simulink model "Simulink_Model"  (R2023a)
settings: Solver=VariableStepAuto  StartTime=0.0  StopTime=10.0  RelTol=1e-3
undefined symbols (not defined in the file or in its folder): aoa, Earth, gustU_pert, gustV_pert, gustW_pert, InConds, mach, rocketAeroDatabase, WGS84
libraries: aerolibatmos2 x2, aerolibwind2 x1, aerolibtransform2 x1
settings Model: Creator=cnsyk  LastModifiedBy=cnsyk

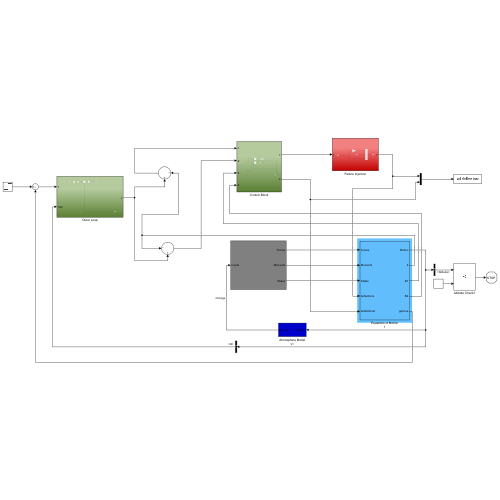
[thumbnail: Simulink's stored preview of the top-level diagram]
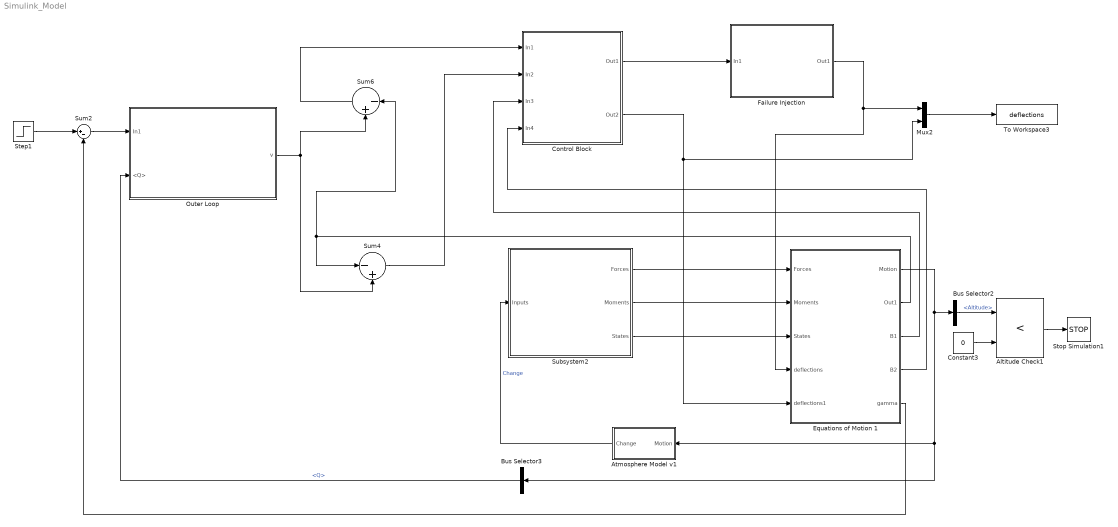
== system Simulink_Model ==
  Altitude Check1 : RelationalOperator  Operator=<  OutDataTypeStr=boolean  RndMeth=Simplest  InputSameDT=off
  Atmosphere Model v1 : Subsystem
  Bus Selector2 : BusSelector  OutputSignals=Altitude
  Bus Selector3 : BusSelector  OutputSignals=Q
  Constant3 : Constant  Value=0
  Control Block : Subsystem
  Equations of Motion 1 : Subsystem
  Failure Injection : Subsystem
  Mux2 : Mux  Inputs=2
  Outer Loop : Subsystem
  Step1 : Step  Time=0  After=deg2rad(80)  SampleTime=0
  Stop Simulation1 : Stop
  Subsystem2 : Subsystem
  Sum2 : Sum  Inputs=|+-
  Sum4 : Sum  Inputs=|-+
  Sum6 : Sum  Inputs=|-+
  To Workspace3 : ToWorkspace  VariableName=deflections  SampleTime=-1
  wires:
  Constant3/1 -> Altitude Check1/2
  Equations of Motion 1/2(Out1) -> Sum4/1, Sum6/1
  Subsystem2/3(States) -> Equations of Motion 1/3(States)
  Subsystem2/2(Moments) -> Equations of Motion 1/2("Moments ")
  Subsystem2/1(Forces) -> Equations of Motion 1/1("Forces ")
  Equations of Motion 1/5(gamma) -> Sum2/2
  Bus Selector2/1 -> Altitude Check1/1  "<Altitude>"
  Altitude Check1/1 -> Stop Simulation1/1
  Step1/1 -> Sum2/1
  Mux2/1 -> To Workspace3/1
  Equations of Motion 1/1(Motion) -> Atmosphere Model v1/1("Motion "), Bus Selector3/1, Bus Selector2/1
  Atmosphere Model v1/1(Change) -> Subsystem2/1("Inputs ")  "Change"
  Control Block/2(Out2) -> Mux2/2, Equations of Motion 1/5(deflections1)
  Sum6/1 -> Control Block/1(In1)
  Sum4/1 -> Control Block/2(In2)
  Equations of Motion 1/3(B1) -> Control Block/3(In3)
  Equations of Motion 1/4(B2) -> Control Block/4(In4)
  Failure Injection/1(Out1) -> Equations of Motion 1/4(deflections), Mux2/1
  Control Block/1(Out1) -> Failure Injection/1(In1)
  Outer Loop/1(v) -> Sum4/2, Sum6/2
  Sum2/1 -> Outer Loop/1(In1)
  Bus Selector3/1 -> Outer Loop/2(<Q>)  "<Q>"

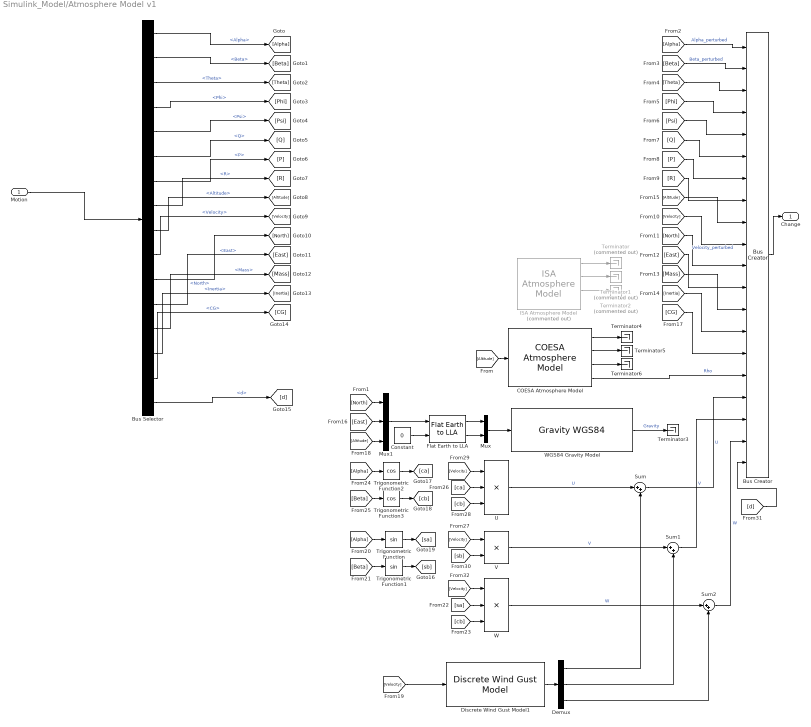
== system Simulink_Model/Atmosphere Model v1 ==
  "Motion " : Inport
  Bus Creator : BusCreator  Inputs=20
  Bus Selector : BusSelector  OutputSignals=Alpha,Beta,Theta,Phi,Psi,Q,P,R,Altitude,Velocity,North,East,Mass,Inertia,CG,d
  COESA Atmosphere Model : aerolibatmos2/COESA Atmosphere Model  units=Metric (MKS)  spec=1976 COESA-extended U.S. Standard Atmosphere  model=Profile  profile_var=High temperature  profile_percent=1%  profile_alt=5 km (16404 ft)  envelope_var=High temperature  envelope_percent=1%  action=Warning
  Constant : Constant  Value=0
  Demux : Demux  Outputs=3
  Discrete Wind Gust Model1 : aerolibwind2/Discrete Wind Gust Model  units=Metric (MKS)  Gx=on  Gy=on  Gz=on  t_0=5  d_m=[120 120 80]  v_m=[gustU_pert gustV_pert gustW_pert]
  Flat Earth to LLA : aerolibtransform2/Flat Earth to LLA  units=Metric (MKS)  ptype=Earth (WGS84)  F=1/298.257223563  R=6378137  refPosPort=off  LL0=[0 10]  psi=0
  ISA Atmosphere Model : aerolibatmos2/ISA Atmosphere Model  Commented=on  custom=off  g=9.80665  gamma=1.4  R=287.0531  L=0.0065  h_trop=11000  h_strat=20000  rho0=1.225  P0=101325  T0=288.15  h0=0
  Mux : Mux  Inputs=2
  Mux1 : Mux  Inputs=3
  Sum : Sum  Inputs=|++
  Sum1 : Sum  Inputs=|++
  Sum2 : Sum  Inputs=|++
  Terminator : Terminator  Commented=on
  Terminator1 : Terminator  Commented=on
  Terminator2 : Terminator  Commented=on
  Terminator{3..6} (4 alike) : Terminator
  Trigonometric Function : Trigonometry
  Trigonometric Function1 : Trigonometry
  Trigonometric Function2 : Trigonometry  Operator=cos
  Trigonometric Function3 : Trigonometry  Operator=cos
  U : Product  Inputs=3
  V : Product
  W : Product  Inputs=3
  "WGS84 Gravity Model  " : GravityWGS84
  Change : Outport  VectorParamsAs1DForOutWhenUnconnected=off
  wires:
  V/1 -> Sum1/1  "V"
  [Q] -> Bus Creator/6
  [ca] -> U/2
  [Phi] -> Bus Creator/4
  [R] -> Bus Creator/8
  [East] -> Bus Creator/12
  Bus Selector/5 -> [Psi]  "<Psi>"
  W/1 -> Sum2/1  "W"
  [Velocity] -> U/1
  [Theta] -> Bus Creator/3
  [sa] -> W/2
  Sum1/1 -> Bus Creator/18  "V"
  [sb] -> V/2
  U/1 -> Sum/1  "U"
  [North] -> Bus Creator/11
  Sum2/1 -> Bus Creator/19  "W"
  [Velocity] -> W/1
  [Altitude] -> Mux1/3
  Trigonometric Function/1 -> [sa]
  Mux/1 -> "WGS84 Gravity Model  "/1
  Bus Selector/7 -> [P]  "<P>"
  [Mass] -> Bus Creator/13
  [cb] -> U/3
  Trigonometric Function2/1 -> [ca]
  [cb] -> W/3
  Demux/2 -> Sum1/2
  [Altitude] -> Bus Creator/9
  Bus Selector/15 -> [CG]  "<CG>"
  ISA Atmosphere Model/2 -> Terminator1/1
  [Beta] -> Trigonometric Function3/1
  Discrete Wind Gust Model1/1 -> Demux/1
  [CG] -> Bus Creator/15
  Bus Selector/1 -> [Alpha]  "<Alpha>"
  [Alpha] -> Trigonometric Function/1
  [Beta] -> Bus Creator/2  "Beta_perturbed"
  Demux/3 -> Sum2/2
  [Beta] -> Trigonometric Function1/1
  "Motion "/1 -> Bus Selector/1
  [Velocity] -> Bus Creator/10  "Velocity_perturbed"
  Bus Selector/8 -> [R]  "<R>"
  Sum/1 -> Bus Creator/17  "U"
  Bus Selector/2 -> [Beta]  "<Beta>"
  Bus Selector/6 -> [Q]  "<Q>"
  "WGS84 Gravity Model  "/1 -> Terminator3/1  "Gravity"
  Mux1/1 -> Flat Earth to LLA/1
  Bus Selector/9 -> [Altitude]  "<Altitude>"
  [P] -> Bus Creator/7
  [East] -> Mux1/2
  [Velocity] -> Discrete Wind Gust Model1/1
  Bus Selector/14 -> [Inertia]  "<Inertia>"
  Bus Selector/10 -> [Velocity]  "<Velocity>"
  Trigonometric Function1/1 -> [sb]
  [Inertia] -> Bus Creator/14
  Bus Selector/11 -> [North]  "<North>"
  Trigonometric Function3/1 -> [cb]
  Bus Selector/4 -> [Phi]  "<Phi>"
  Bus Selector/12 -> [East]  "<East>"
  Bus Selector/3 -> [Theta]  "<Theta>"
  [Alpha] -> Bus Creator/1  "Alpha_perturbed"
  [Psi] -> Bus Creator/5
  Constant/1 -> Flat Earth to LLA/2
  [North] -> Mux1/1
  Bus Creator/1 -> Change/1
  ISA Atmosphere Model/1 -> Terminator/1
  Flat Earth to LLA/1 -> Mux/1
  Demux/1 -> Sum/2
  Bus Selector/13 -> [Mass]  "<Mass>"
  [Velocity] -> V/1
  ISA Atmosphere Model/3 -> Terminator2/1
  [Alpha] -> Trigonometric Function2/1
  Flat Earth to LLA/2 -> Mux/2
  [Altitude] -> COESA Atmosphere Model/1
  COESA Atmosphere Model/1 -> Terminator4/1
  COESA Atmosphere Model/2 -> Terminator5/1
  COESA Atmosphere Model/3 -> Terminator6/1
  COESA Atmosphere Model/4 -> Bus Creator/16  "Rho"
  Bus Selector/16 -> [d]  "<d>"
  [d] -> Bus Creator/20

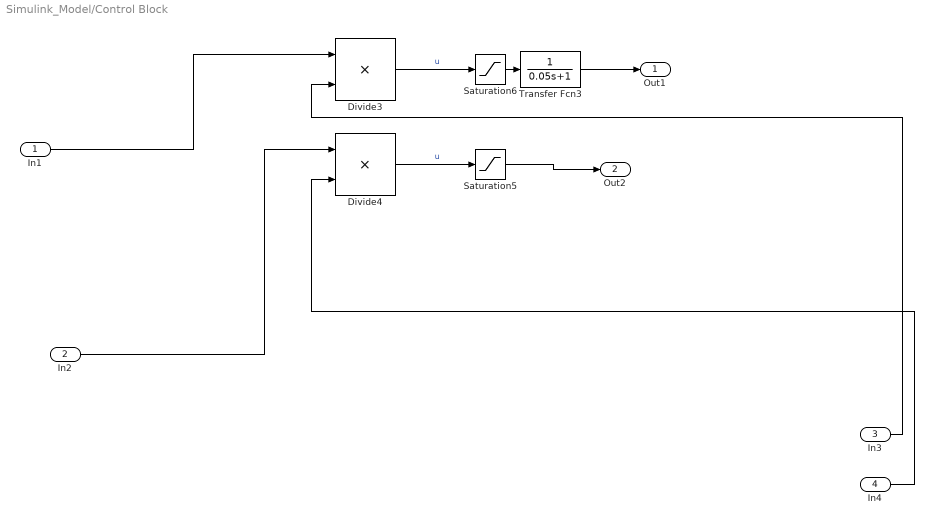
== system Simulink_Model/Control Block ==
  In1 : Inport
  In2 : Inport  Port=2
  In3 : Inport  Port=3
  In4 : Inport  Port=4
  Divide3 : Product  Inputs=**
  Divide4 : Product  Inputs=**
  Saturation5 : Saturate  UpperLimit=deg2rad(5)  LowerLimit=-deg2rad(5)
  Saturation6 : Saturate  UpperLimit=deg2rad(5)  LowerLimit=-deg2rad(5)
  Transfer Fcn3 : TransferFcn  Denominator=[0.05 1]
  Out1 : Outport
  Out2 : Outport  Port=2
  wires:
  In3/1 -> Divide3/2
  In4/1 -> Divide4/2
  Saturation5/1 -> Out2/1
  Saturation6/1 -> Transfer Fcn3/1
  Divide3/1 -> Saturation6/1  "u"
  Divide4/1 -> Saturation5/1  "u"
  In2/1 -> Divide4/1
  In1/1 -> Divide3/1
  Transfer Fcn3/1 -> Out1/1

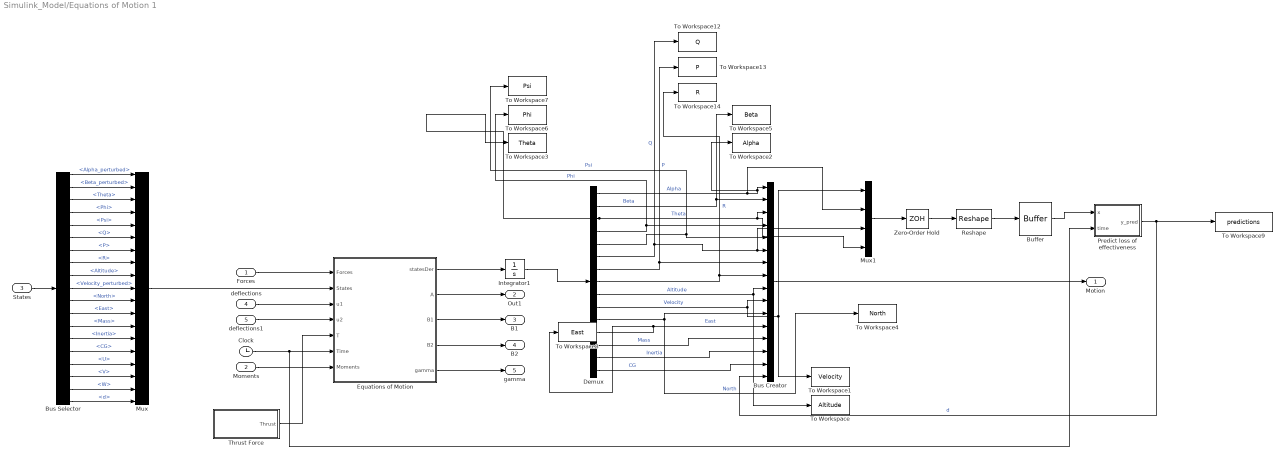
== system Simulink_Model/Equations of Motion 1 ==
  "Forces " : Inport
  "Moments " : Inport  Port=2
  States : Inport  Port=3
  deflections : Inport  Port=4
  deflections1 : Inport  Port=5
  Buffer : Buffer  N=20  V=19  OutputFrames=off
  Bus Creator : BusCreator  Inputs=16
  Bus Selector : BusSelector  OutputSignals=Alpha_perturbed,Beta_perturbed,Theta,Phi,Psi,Q,P,R,Altitude,Velocity_perturbed,North,East,Mass,Inertia,CG,U,V,W,d
  Clock : Clock
  Demux : Demux  Outputs=15
  Equations of Motion : MATLAB Function  TreatAsAtomicUnit=on
  Integrator1 : Integrator  InitialCondition=InConds
  Mux : Mux  Inputs=19
  Mux1 : Mux
  Predict loss of effectiveness : MATLAB Function  TreatAsAtomicUnit=on
  Reshape : Reshape  OutputDimensionality=Customize  OutputDimensions=[1,4]
  "Thrust Force " : Subsystem
  To Workspace : ToWorkspace  VariableName=Altitude  SampleTime=-1
  To Workspace1 : ToWorkspace  VariableName=Velocity  SampleTime=-1
  To Workspace12 : ToWorkspace  VariableName=Q  SampleTime=-1
  To Workspace13 : ToWorkspace  VariableName=P  SampleTime=-1
  To Workspace14 : ToWorkspace  VariableName=R  SampleTime=-1
  To Workspace2 : ToWorkspace  VariableName=Alpha  SampleTime=-1
  To Workspace3 : ToWorkspace  VariableName=Theta  SampleTime=-1
  To Workspace4 : ToWorkspace  VariableName=North  SampleTime=-1
  To Workspace5 : ToWorkspace  VariableName=Beta  SampleTime=-1
  To Workspace6 : ToWorkspace  VariableName=Phi  SampleTime=-1
  To Workspace7 : ToWorkspace  VariableName=Psi  SampleTime=-1
  To Workspace8 : ToWorkspace  VariableName=East  SampleTime=-1
  To Workspace9 : ToWorkspace  VariableName=predictions  SampleTime=-1
  Zero-Order Hold : ZeroOrderHold  SampleTime=-1
  Motion : Outport  VectorParamsAs1DForOutWhenUnconnected=off
  Out1 : Outport  Port=2
  B1 : Outport  Port=3
  B2 : Outport  Port=4
  gamma : Outport  Port=5
  wires:
  "Moments "/1 -> Equations of Motion/7(Moments)
  "Forces "/1 -> Equations of Motion/1(Forces)
  Demux/10 -> Bus Creator/10, To Workspace1/1, Mux1/1  "Velocity"
  Demux/9 -> Bus Creator/9, To Workspace/1  "Altitude"
  Demux/8 -> To Workspace14/1, Bus Creator/8  "R"
  Demux/7 -> To Workspace13/1, Bus Creator/7  "P"
  Demux/6 -> Mux1/3, Bus Creator/6, To Workspace12/1  "Q"
  Demux/5 -> To Workspace7/1, Bus Creator/5  "Psi"
  Demux/4 -> To Workspace6/1, Bus Creator/4  "Phi"
  Demux/3 -> Mux1/4, Bus Creator/3, To Workspace3/1  "Theta"
  Bus Creator/1 -> Motion/1
  Demux/11 -> To Workspace4/1, Bus Creator/11  "North"
  Demux/12 -> To Workspace8/1, Bus Creator/12  "East"
  Demux/13 -> Bus Creator/13  "Mass"
  Demux/14 -> Bus Creator/14  "Inertia"
  Demux/15 -> Bus Creator/15  "CG"
  States/1 -> Bus Selector/1
  Mux/1 -> Equations of Motion/2(States)
  Clock/1 -> Equations of Motion/6(Time), Predict loss of effectiveness/2(time)
  Bus Selector/1 -> Mux/1  "<Alpha_perturbed>"
  Bus Selector/5 -> Mux/5  "<Psi>"
  Bus Selector/4 -> Mux/4  "<Phi>"
  Bus Selector/3 -> Mux/3  "<Theta>"
  Bus Selector/2 -> Mux/2  "<Beta_perturbed>"
  Demux/1 -> Mux1/2, Bus Creator/1, To Workspace2/1  "Alpha"
  Demux/2 -> To Workspace5/1, Bus Creator/2  "Beta"
  Bus Selector/6 -> Mux/6  "<Q>"
  Bus Selector/7 -> Mux/7  "<P>"
  Bus Selector/8 -> Mux/8  "<R>"
  Bus Selector/9 -> Mux/9  "<Altitude>"
  Bus Selector/14 -> Mux/14  "<Inertia>"
  Bus Selector/13 -> Mux/13  "<Mass>"
  Bus Selector/12 -> Mux/12  "<East>"
  Bus Selector/11 -> Mux/11  "<North>"
  Bus Selector/10 -> Mux/10  "<Velocity_perturbed>"
  Bus Selector/15 -> Mux/15  "<CG>"
  Bus Selector/17 -> Mux/17  "<V>"
  Bus Selector/16 -> Mux/16  "<U>"
  Bus Selector/18 -> Mux/18  "<W>"
  deflections/1 -> Equations of Motion/3(u1)
  Equations of Motion/3(B1) -> B1/1
  Equations of Motion/2(A) -> Out1/1
  "Thrust Force "/1(Thrust) -> Equations of Motion/5(T)
  Equations of Motion/5(gamma) -> gamma/1
  Integrator1/1 -> Demux/1
  deflections1/1 -> Equations of Motion/4(u2)
  Equations of Motion/4(B2) -> B2/1
  Equations of Motion/1(statesDer) -> Integrator1/1
  Reshape/1 -> Buffer/1
  Buffer/1 -> Predict loss of effectiveness/1(x)
  Predict loss of effectiveness/1(y_pred) -> To Workspace9/1, Bus Creator/16  "d"
  Mux1/1 -> Zero-Order Hold/1
  Zero-Order Hold/1 -> Reshape/1
  Bus Selector/19 -> Mux/19  "<d>"

== system Simulink_Model/Failure Injection ==
  In1 : Inport
  Clock2 : Clock
  Gain4 : Gain
  Switch2 : Switch  Criteria=u2 > Threshold  Threshold=6  SaturateOnIntegerOverflow=off  InputSameDT=off
  Out1 : Outport
  wires:
  In1/1 -> Switch2/3, Gain4/1
  Gain4/1 -> Switch2/1
  Clock2/1 -> Switch2/2
  Switch2/1 -> Out1/1

== system Simulink_Model/Outer Loop ==
  In1 : Inport
  <Q> : Inport  Port=2
  Delay2 : Delay  DelayLength=3  InitialCondition=0
  Gain2 : Gain  Gain=5
  Gain3 : Gain  Gain=10
  Saturation4 : Saturate  UpperLimit=deg2rad(5)  LowerLimit=-deg2rad(5)
  Sum5 : Sum  Inputs=|+-
  v : Outport
  wires:
  Delay2/1 -> Saturation4/1
  Gain3/1 -> v/1  "v"
  Gain2/1 -> Delay2/1
  <Q>/1 -> Sum5/2
  In1/1 -> Gain2/1
  Sum5/1 -> Gain3/1
  Saturation4/1 -> Sum5/1

== system Simulink_Model/Subsystem2 ==
  "Inputs " : Inport
  Moment Calculation : Subsystem
  Mux : Mux  Inputs=3
  Mux1 : Mux  Inputs=3
  Subsystem1 : Subsystem
  Forces : Outport  VectorParamsAs1DForOutWhenUnconnected=off
  Moments : Outport  Port=2  VectorParamsAs1DForOutWhenUnconnected=off
  States : Outport  Port=3  VectorParamsAs1DForOutWhenUnconnected=off
  wires:
  "Inputs "/1 -> Subsystem1/1("Inputs "), States/1, Moment Calculation/1("Inputs ")
  Moment Calculation/1("MCm ") -> Mux1/1
  Moment Calculation/2(MCl) -> Mux1/2
  Subsystem1/3(FCY) -> Mux/3
  Mux/1 -> Forces/1
  Subsystem1/1(FCL) -> Mux/1
  Mux1/1 -> Moments/1
  Subsystem1/2(FCD) -> Mux/2
  Moment Calculation/3(MCn) -> Mux1/3

== system Simulink_Model/Equations of Motion 1/Thrust Force  ==
  Clock : Clock
  If : If  IfExpression=u1 < 33
  If Action Subsystem : Subsystem  TreatAsAtomicUnit=on
  If Action Subsystem1 : Subsystem  TreatAsAtomicUnit=on
  Scope : Scope
  Sum : Sum  Inputs=+|+
  To Workspace : ToWorkspace  VariableName=thrust  SampleTime=-1
  Thrust : Outport  VectorParamsAs1DForOutWhenUnconnected=off
  wires:
  Sum/1 -> To Workspace/1, Thrust/1
  Clock/1 -> If Action Subsystem1/1(Time), If Action Subsystem/1(Time), If/1
  If/1 -> If Action Subsystem/Action
  If Action Subsystem/1(Thrust) -> Scope/1, Sum/1
  If/2 -> If Action Subsystem1/Action
  If Action Subsystem1/1(Thrust) -> Sum/2

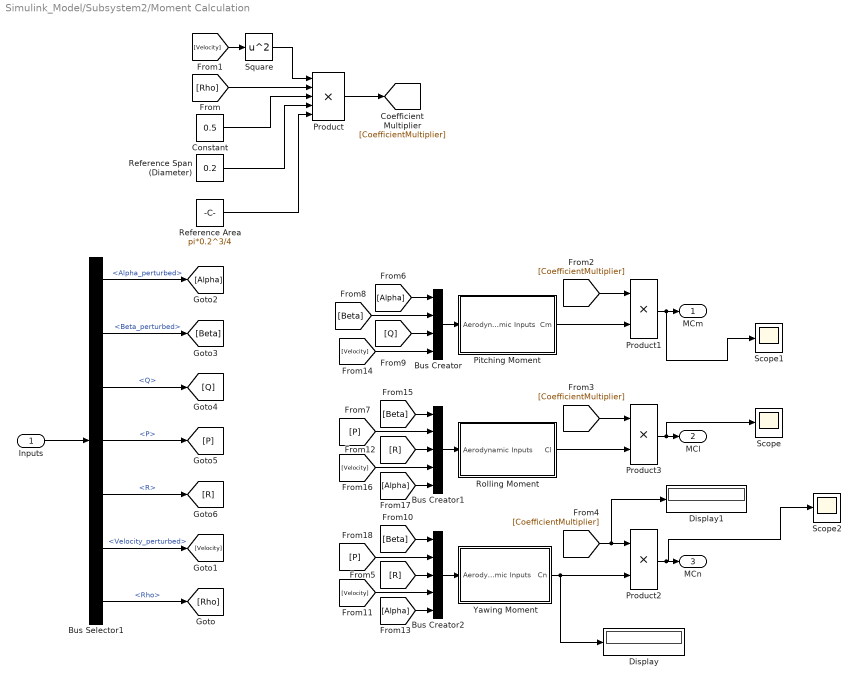
== system Simulink_Model/Subsystem2/Moment Calculation ==
  "Inputs " : Inport
  Bus Creator : BusCreator  Inputs=4
  Bus Creator1 : BusCreator  Inputs=5
  Bus Creator2 : BusCreator  Inputs=5
  Bus Selector1 : BusSelector  OutputSignals=Alpha_perturbed,Beta_perturbed,Q,P,R,Velocity_perturbed,Rho
  Constant : Constant  Value=0.5
  Display : Display
  Display1 : Display
  Pitching Moment : Subsystem
  Product : Product  Inputs=5
  Product1 : Product
  Product2 : Product
  Product3 : Product
  Reference Area : Constant  Value=pi*0.2^3/4
  Reference Span (Diameter) : Constant  Value=0.2
  Rolling Moment : Subsystem
  Scope : Scope
  Scope1 : Scope
  Scope2 : Scope
  Square : Math  Operator=square  SignedPower=on
  Yawing Moment : Subsystem
  "MCm " : Outport  VectorParamsAs1DForOutWhenUnconnected=off
  MCl : Outport  Port=2  VectorParamsAs1DForOutWhenUnconnected=off
  MCn : Outport  Port=3  VectorParamsAs1DForOutWhenUnconnected=off
  wires:
  Bus Selector1/4 -> [P]  "<P>"
  Bus Selector1/3 -> [Q]  "<Q>"
  Bus Selector1/5 -> [R]  "<R>"
  Bus Selector1/1 -> [Alpha]  "<Alpha_perturbed>"
  Bus Selector1/2 -> [Beta]  "<Beta_perturbed>"
  Product1/1 -> Scope1/1, "MCm "/1
  Product/1 -> [CoefficientMultiplier]
  [Velocity] -> Square/1
  [CoefficientMultiplier] -> Product1/1
  Reference Span (Diameter)/1 -> Product/4
  Bus Selector1/7 -> [Rho]  "<Rho>"
  Product3/1 -> Scope/1, MCl/1
  [CoefficientMultiplier] -> Display1/1, Product2/1
  [CoefficientMultiplier] -> Product3/1
  Bus Selector1/6 -> [Velocity]  "<Velocity_perturbed>"
  [Rho] -> Product/2
  "Inputs "/1 -> Bus Selector1/1
  Square/1 -> Product/1
  Constant/1 -> Product/3
  Bus Creator/1 -> Pitching Moment/1(Aerodynamic Inputs)
  [Alpha] -> Bus Creator/1
  [Q] -> Bus Creator/3
  [Beta] -> Bus Creator/2
  Bus Creator1/1 -> Rolling Moment/1(Aerodynamic Inputs)
  [Beta] -> Bus Creator1/1
  [P] -> Bus Creator1/2
  [R] -> Bus Creator1/3
  [Velocity] -> Bus Creator1/4
  Bus Creator2/1 -> Yawing Moment/1(Aerodynamic Inputs)
  Yawing Moment/1(Cn) -> Display/1, Product2/2
  [Velocity] -> Bus Creator/4
  [Alpha] -> Bus Creator1/5
  [P] -> Bus Creator2/2
  [Velocity] -> Bus Creator2/4
  [R] -> Bus Creator2/3
  [Beta] -> Bus Creator2/1
  [Alpha] -> Bus Creator2/5
  Reference Area/1 -> Product/5
  Pitching Moment/1(Cm) -> Product1/2
  Rolling Moment/1(Cl) -> Product3/2
  Product2/1 -> Scope2/1, MCn/1

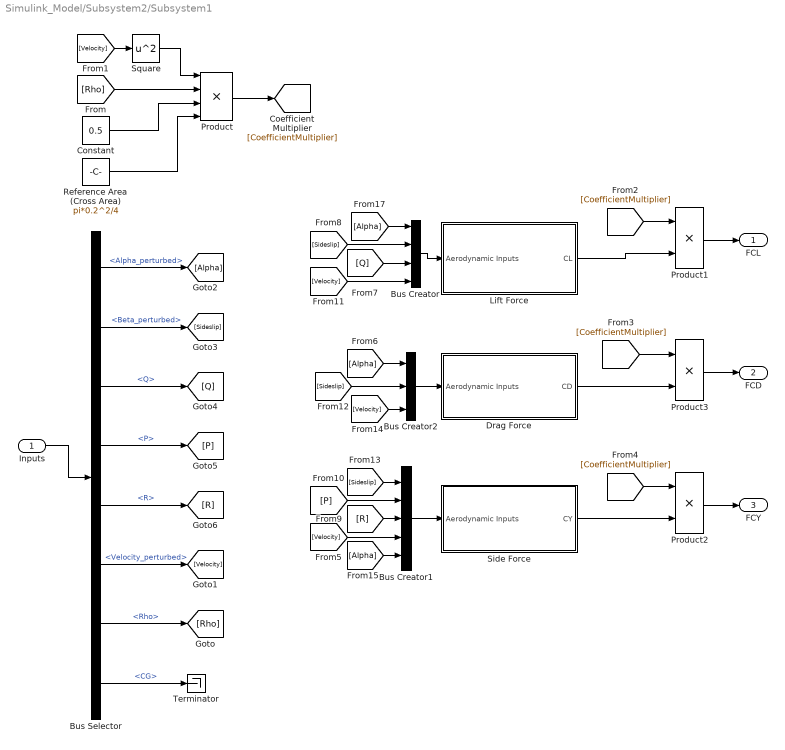
== system Simulink_Model/Subsystem2/Subsystem1 ==
  "Inputs " : Inport
  Bus Creator : BusCreator  Inputs=4
  Bus Creator1 : BusCreator  Inputs=5
  Bus Creator2 : BusCreator  Inputs=3
  Bus Selector : BusSelector  OutputSignals=Alpha_perturbed,Beta_perturbed,Q,P,R,Velocity_perturbed,Rho,CG
  Constant : Constant  Value=0.5
  Drag Force : Subsystem
  "Lift Force " : Subsystem
  Product : Product  Inputs=4
  Product1 : Product
  Product2 : Product
  Product3 : Product
  Reference Area (Cross Area) : Constant  Value=pi*0.2^2/4
  Side Force : Subsystem
  Square : Math  Operator=square  SignedPower=on
  Terminator : Terminator
  FCL : Outport  VectorParamsAs1DForOutWhenUnconnected=off
  FCD : Outport  Port=2  VectorParamsAs1DForOutWhenUnconnected=off
  FCY : Outport  Port=3  VectorParamsAs1DForOutWhenUnconnected=off
  wires:
  Product1/1 -> FCL/1
  Bus Selector/7 -> [Rho]  "<Rho>"
  Drag Force/1(CD) -> Product3/2
  Bus Creator/1 -> "Lift Force "/1(Aerodynamic Inputs)
  [Rho] -> Product/2
  Side Force/1(CY) -> Product2/2
  Bus Selector/5 -> [R]  "<R>"
  Bus Creator1/1 -> Side Force/1(Aerodynamic Inputs)
  [Sideslip] -> Bus Creator1/1
  "Lift Force "/1(CL) -> Product1/2
  [Sideslip] -> Bus Creator/2
  [Q] -> Bus Creator/3
  [Velocity] -> Bus Creator2/3
  [Alpha] -> Bus Creator2/1
  Product/1 -> [CoefficientMultiplier]
  [Sideslip] -> Bus Creator2/2
  [Velocity] -> Bus Creator1/4
  Bus Selector/2 -> [Sideslip]  "<Beta_perturbed>"
  Bus Selector/4 -> [P]  "<P>"
  [Velocity] -> Bus Creator/4
  Reference Area (Cross Area)/1 -> Product/4
  [P] -> Bus Creator1/2
  "Inputs "/1 -> Bus Selector/1
  [Alpha] -> Bus Creator1/5
  Product3/1 -> FCD/1
  [Alpha] -> Bus Creator/1
  Constant/1 -> Product/3
  Bus Selector/1 -> [Alpha]  "<Alpha_perturbed>"
  [R] -> Bus Creator1/3
  Product2/1 -> FCY/1
  [CoefficientMultiplier] -> Product3/1
  [Velocity] -> Square/1
  Bus Selector/3 -> [Q]  "<Q>"
  [CoefficientMultiplier] -> Product2/1
  Bus Creator2/1 -> Drag Force/1(Aerodynamic Inputs)
  Bus Selector/8 -> Terminator/1  "<CG>"
  [CoefficientMultiplier] -> Product1/1
  Bus Selector/6 -> [Velocity]  "<Velocity_perturbed>"
  Square/1 -> Product/1

== system Simulink_Model/Equations of Motion 1/Thrust Force /If Action Subsystem ==
  Time : Inport
  Action Port : ActionPort
  1-D Lookup Table : Lookup_n-D  NumberOfTableDimensions=1  BreakpointsForDimension1=rocketAeroDatabase.Thrust(1:end,1)  Table=rocketAeroDatabase.Thrust(1:end,2)  UseLastTableValue=on  InternalRulePriority=Speed  RndMeth=Simplest
  Thrust : Outport  VectorParamsAs1DForOutWhenUnconnected=off
  wires:
  Time/1 -> 1-D Lookup Table/1
  1-D Lookup Table/1 -> Thrust/1

== system Simulink_Model/Equations of Motion 1/Thrust Force /If Action Subsystem1 ==
  Time : Inport
  Action Port : ActionPort
  1-D Lookup Table : Lookup_n-D  NumberOfTableDimensions=1  BreakpointsForDimension1=rocketAeroDatabase.Thrust(1:end,1)  Table=rocketAeroDatabase.Thrust(1:end,2)  UseLastTableValue=on  InternalRulePriority=Speed  RndMeth=Simplest
  Gain1 : Gain  Gain=0
  Thrust : Outport  VectorParamsAs1DForOutWhenUnconnected=off
  wires:
  Time/1 -> 1-D Lookup Table/1
  1-D Lookup Table/1 -> Gain1/1
  Gain1/1 -> Thrust/1

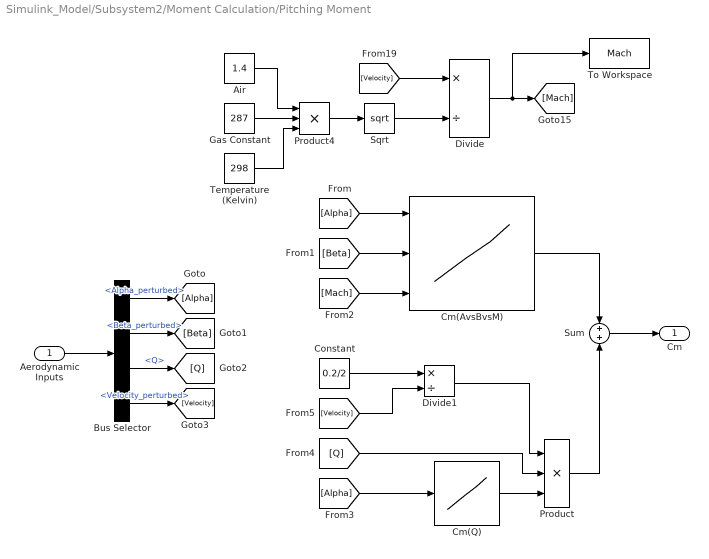
== system Simulink_Model/Subsystem2/Moment Calculation/Pitching Moment ==
  Aerodynamic Inputs : Inport
  Air : Constant  Value=1.4
  Bus Selector : BusSelector  OutputSignals=Alpha_perturbed,Beta_perturbed,Q,Velocity_perturbed
  Cm(AvsBvsM) : Lookup_n-D  NumberOfTableDimensions=3  BreakpointsForDimension1=[deg2rad(aoa(1)), deg2rad(aoa(2)), deg2rad(aoa(3)), deg2rad(aoa(4)), deg2rad(aoa(5))]  BreakpointsForDimension2=[deg2rad(ss(1)), deg2rad(ss(2)), deg2rad(ss(3)), deg2rad(ss(4))]  BreakpointsForDimension3=[mach(1), mach(2), mach(3), mach(4), mach(5)]  Table=rocketAeroDatabase.pitch.Cm  InternalRulePriority=Speed  RndMeth=Simplest
      settings: InputPortMap=u0,u1,u2
  Cm(Q) : Lookup_n-D  NumberOfTableDimensions=1  BreakpointsForDimension1=[-5 5]  Table=[-2400 -2400]  InternalRulePriority=Speed  RndMeth=Simplest
  Constant : Constant  Value=0.2/2
  Divide : Product  Inputs=*/
  Divide1 : Product  Inputs=*/
  Gas Constant : Constant  Value=287
  Product : Product  Inputs=3
  Product4 : Product  Inputs=3
  Sqrt : Sqrt
  Sum : Sum  Inputs=+|+
  Temperature (Kelvin) : Constant  Value=298
  To Workspace : ToWorkspace  VariableName=Mach  SampleTime=-1
  Cm : Outport  VectorParamsAs1DForOutWhenUnconnected=off
  wires:
  Bus Selector/4 -> [Velocity]  "<Velocity_perturbed>"
  [Mach] -> Cm(AvsBvsM)/3
  [Alpha] -> Cm(AvsBvsM)/1
  Bus Selector/1 -> [Alpha]  "<Alpha_perturbed>"
  Aerodynamic Inputs/1 -> Bus Selector/1
  Bus Selector/2 -> [Beta]  "<Beta_perturbed>"
  Bus Selector/3 -> [Q]  "<Q>"
  Sum/1 -> Cm/1
  Product4/1 -> Sqrt/1
  Air/1 -> Product4/1
  Temperature (Kelvin)/1 -> Product4/3
  Gas Constant/1 -> Product4/2
  Sqrt/1 -> Divide/2
  Divide/1 -> To Workspace/1, [Mach]
  [Velocity] -> Divide/1
  [Alpha] -> Cm(Q)/1
  Constant/1 -> Divide1/1
  Divide1/1 -> Product/1
  [Q] -> Product/2
  Cm(Q)/1 -> Product/3
  [Velocity] -> Divide1/2
  Product/1 -> Sum/2
  [Beta] -> Cm(AvsBvsM)/2
  Cm(AvsBvsM)/1 -> Sum/1

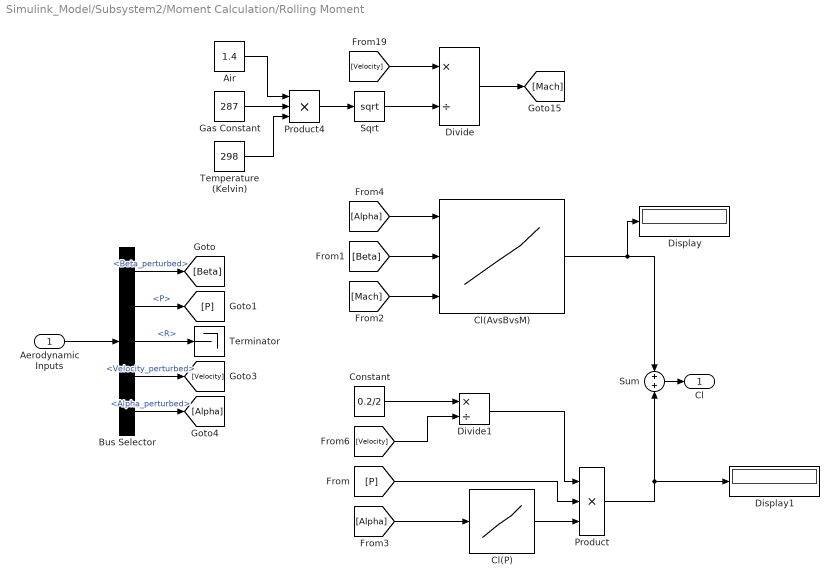
== system Simulink_Model/Subsystem2/Moment Calculation/Rolling Moment ==
  Aerodynamic Inputs : Inport
  Air : Constant  Value=1.4
  Bus Selector : BusSelector  OutputSignals=Beta_perturbed,P,R,Velocity_perturbed,Alpha_perturbed
  Cl(AvsBvsM) : Lookup_n-D  NumberOfTableDimensions=3  BreakpointsForDimension1=[deg2rad(aoa(1)), deg2rad(aoa(2)), deg2rad(aoa(3)), deg2rad(aoa(4)), deg2rad(aoa(5))]  BreakpointsForDimension2=[deg2rad(ss(1)), deg2rad(ss(2)), deg2rad(ss(3)), deg2rad(ss(4))]  BreakpointsForDimension3=[mach(1), mach(2), mach(3), mach(4), mach(5)]  Table=-rocketAeroDatabase.roll.Croll  InternalRulePriority=Speed  RndMeth=Simplest
      settings: InputPortMap=u0,u1,u2
  Cl(P) : Lookup_n-D  NumberOfTableDimensions=1  BreakpointsForDimension1=[-5 5]  Table=[-45 -45]  InternalRulePriority=Speed  RndMeth=Simplest
  Constant : Constant  Value=0.2/2
  Display : Display
  Display1 : Display
  Divide : Product  Inputs=*/
  Divide1 : Product  Inputs=*/
  Gas Constant : Constant  Value=287
  Product : Product  Inputs=3
  Product4 : Product  Inputs=3
  Sqrt : Sqrt
  Sum : Sum  Inputs=+|+
  Temperature (Kelvin) : Constant  Value=298
  Terminator : Terminator
  Cl : Outport  VectorParamsAs1DForOutWhenUnconnected=off
  wires:
  Cl(AvsBvsM)/1 -> Display/1, Sum/1
  Aerodynamic Inputs/1 -> Bus Selector/1
  [Beta] -> Cl(AvsBvsM)/2
  [Mach] -> Cl(AvsBvsM)/3
  Bus Selector/1 -> [Beta]  "<Beta_perturbed>"
  Bus Selector/2 -> [P]  "<P>"
  Bus Selector/3 -> Terminator/1  "<R>"
  Bus Selector/4 -> [Velocity]  "<Velocity_perturbed>"
  Product4/1 -> Sqrt/1
  Air/1 -> Product4/1
  Temperature (Kelvin)/1 -> Product4/3
  Gas Constant/1 -> Product4/2
  Sqrt/1 -> Divide/2
  Divide/1 -> [Mach]
  [Velocity] -> Divide/1
  Bus Selector/5 -> [Alpha]  "<Alpha_perturbed>"
  [Alpha] -> Cl(AvsBvsM)/1
  [Alpha] -> Cl(P)/1
  Constant/1 -> Divide1/1
  Divide1/1 -> Product/1
  [P] -> Product/2
  Cl(P)/1 -> Product/3
  [Velocity] -> Divide1/2
  Product/1 -> Sum/2, Display1/1
  Sum/1 -> Cl/1

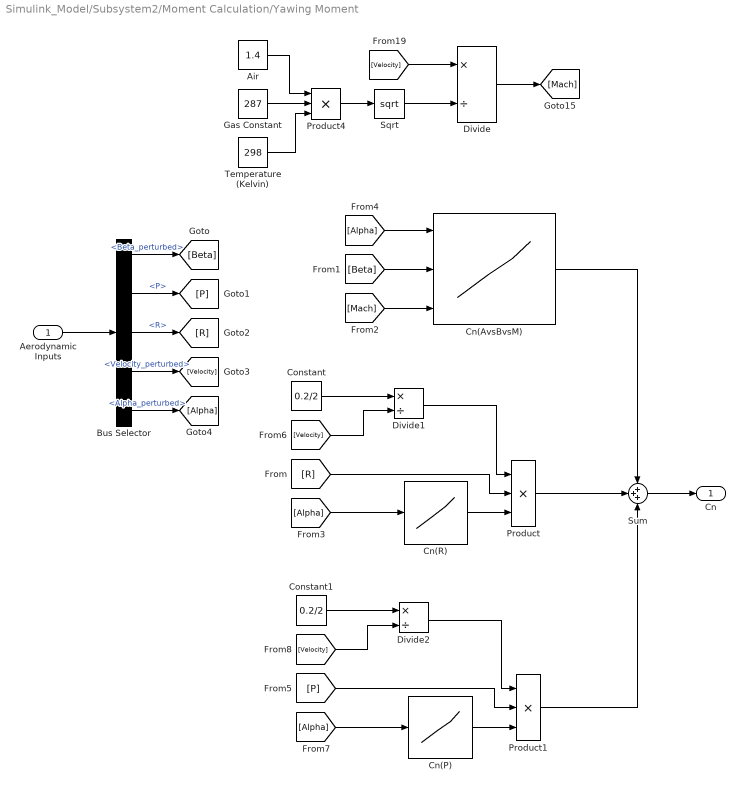
== system Simulink_Model/Subsystem2/Moment Calculation/Yawing Moment ==
  Aerodynamic Inputs : Inport
  Air : Constant  Value=1.4
  Bus Selector : BusSelector  OutputSignals=Beta_perturbed,P,R,Velocity_perturbed,Alpha_perturbed
  Cn(AvsBvsM) : Lookup_n-D  NumberOfTableDimensions=3  BreakpointsForDimension1=[deg2rad(aoa(1)), deg2rad(aoa(2)), deg2rad(aoa(3)), deg2rad(aoa(4)), deg2rad(aoa(5))]  BreakpointsForDimension2=[deg2rad(ss(1)), deg2rad(ss(2)), deg2rad(ss(3)), deg2rad(ss(4))]  BreakpointsForDimension3=[mach(1), mach(2), mach(3), mach(4), mach(5)]  Table=-rocketAeroDatabase.yaw.Cyaw  InternalRulePriority=Speed  RndMeth=Simplest
      settings: InputPortMap=u0,u1,u2
  Cn(P) : Lookup_n-D  NumberOfTableDimensions=1  BreakpointsForDimension1=[-5 5]  Table=[-3000 -3000]  InternalRulePriority=Speed  RndMeth=Simplest
  Cn(R) : Lookup_n-D  NumberOfTableDimensions=1  BreakpointsForDimension1=[-5 5]  Table=[-65 -65]  InternalRulePriority=Speed  RndMeth=Simplest
  Constant : Constant  Value=0.2/2
  Constant1 : Constant  Value=0.2/2
  Divide : Product  Inputs=*/
  Divide1 : Product  Inputs=*/
  Divide2 : Product  Inputs=*/
  Gas Constant : Constant  Value=287
  Product : Product  Inputs=3
  Product1 : Product  Inputs=3
  Product4 : Product  Inputs=3
  Sqrt : Sqrt
  Sum : Sum  Inputs=+++
  Temperature (Kelvin) : Constant  Value=298
  Cn : Outport  VectorParamsAs1DForOutWhenUnconnected=off
  wires:
  Bus Selector/3 -> [R]  "<R>"
  Bus Selector/4 -> [Velocity]  "<Velocity_perturbed>"
  Bus Selector/1 -> [Beta]  "<Beta_perturbed>"
  Bus Selector/2 -> [P]  "<P>"
  Sum/1 -> Cn/1
  Aerodynamic Inputs/1 -> Bus Selector/1
  Product4/1 -> Sqrt/1
  Air/1 -> Product4/1
  Temperature (Kelvin)/1 -> Product4/3
  Gas Constant/1 -> Product4/2
  Sqrt/1 -> Divide/2
  Divide/1 -> [Mach]
  [Velocity] -> Divide/1
  [Beta] -> Cn(AvsBvsM)/2
  [Mach] -> Cn(AvsBvsM)/3
  [Alpha] -> Cn(AvsBvsM)/1
  Cn(AvsBvsM)/1 -> Sum/1
  Bus Selector/5 -> [Alpha]  "<Alpha_perturbed>"
  [Alpha] -> Cn(R)/1
  Constant/1 -> Divide1/1
  Divide1/1 -> Product/1
  [R] -> Product/2
  Cn(R)/1 -> Product/3
  [Velocity] -> Divide1/2
  Product/1 -> Sum/2
  [P] -> Product1/2
  Cn(P)/1 -> Product1/3
  [Velocity] -> Divide2/2
  [Alpha] -> Cn(P)/1
  Divide2/1 -> Product1/1
  Constant1/1 -> Divide2/1
  Product1/1 -> Sum/3

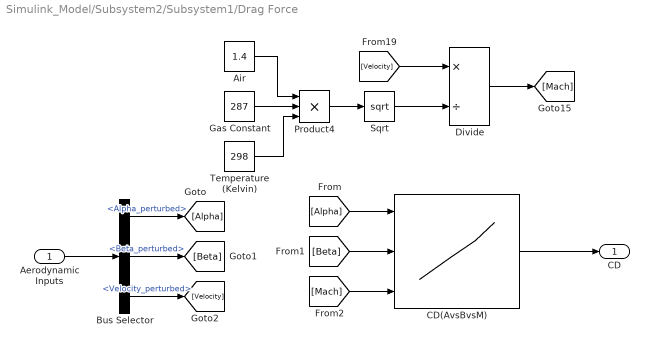
== system Simulink_Model/Subsystem2/Subsystem1/Drag Force ==
  Aerodynamic Inputs : Inport
  Air : Constant  Value=1.4
  Bus Selector : BusSelector  OutputSignals=Alpha_perturbed,Beta_perturbed,Velocity_perturbed
  CD(AvsBvsM) : Lookup_n-D  NumberOfTableDimensions=3  BreakpointsForDimension1=[deg2rad(aoa(1)), deg2rad(aoa(2)), deg2rad(aoa(3)), deg2rad(aoa(4)), deg2rad(aoa(5))]  BreakpointsForDimension2=[deg2rad(ss(1)), deg2rad(ss(2)), deg2rad(ss(3)), deg2rad(ss(4))]  BreakpointsForDimension3=[mach(1), mach(2), mach(3), mach(4), mach(5)]  Table=rocketAeroDatabase.drag.CD  InternalRulePriority=Speed  RndMeth=Simplest
      settings: InputPortMap=u0,u1,u2
  Divide : Product  Inputs=*/
  Gas Constant : Constant  Value=287
  Product4 : Product  Inputs=3
  Sqrt : Sqrt
  Temperature (Kelvin) : Constant  Value=298
  CD : Outport  VectorParamsAs1DForOutWhenUnconnected=off
  wires:
  [Mach] -> CD(AvsBvsM)/3
  CD(AvsBvsM)/1 -> CD/1
  [Alpha] -> CD(AvsBvsM)/1
  [Beta] -> CD(AvsBvsM)/2
  Aerodynamic Inputs/1 -> Bus Selector/1
  Bus Selector/1 -> [Alpha]  "<Alpha_perturbed>"
  Bus Selector/2 -> [Beta]  "<Beta_perturbed>"
  Bus Selector/3 -> [Velocity]  "<Velocity_perturbed>"
  Product4/1 -> Sqrt/1
  Air/1 -> Product4/1
  Temperature (Kelvin)/1 -> Product4/3
  Gas Constant/1 -> Product4/2
  Sqrt/1 -> Divide/2
  Divide/1 -> [Mach]
  [Velocity] -> Divide/1

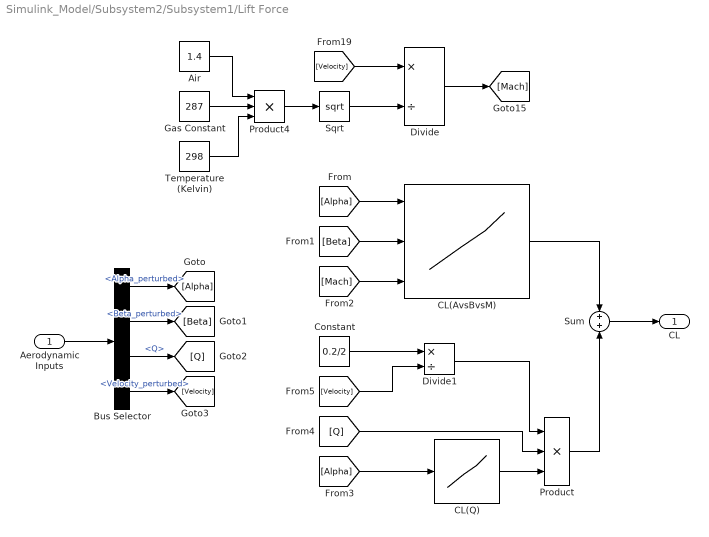
== system Simulink_Model/Subsystem2/Subsystem1/Lift Force  ==
  Aerodynamic Inputs : Inport
  Air : Constant  Value=1.4
  Bus Selector : BusSelector  OutputSignals=Alpha_perturbed,Beta_perturbed,Q,Velocity_perturbed
  CL(AvsBvsM) : Lookup_n-D  NumberOfTableDimensions=3  BreakpointsForDimension1=[deg2rad(aoa(1)), deg2rad(aoa(2)), deg2rad(aoa(3)), deg2rad(aoa(4)), deg2rad(aoa(5))]  BreakpointsForDimension2=[deg2rad(ss(1)), deg2rad(ss(2)), deg2rad(ss(3)), deg2rad(ss(4))]  BreakpointsForDimension3=[mach(1), mach(2), mach(3), mach(4), mach(5)]  Table=rocketAeroDatabase.lift.CL  InternalRulePriority=Speed  RndMeth=Simplest
      settings: InputPortMap=u0,u1,u2
  CL(Q) : Lookup_n-D  NumberOfTableDimensions=1  BreakpointsForDimension1=[-5 5]  Table=[0 0]  InternalRulePriority=Speed  RndMeth=Simplest
  Constant : Constant  Value=0.2/2
  Divide : Product  Inputs=*/
  Divide1 : Product  Inputs=*/
  Gas Constant : Constant  Value=287
  Product : Product  Inputs=3
  Product4 : Product  Inputs=3
  Sqrt : Sqrt
  Sum : Sum  Inputs=+|+
  Temperature (Kelvin) : Constant  Value=298
  CL : Outport  VectorParamsAs1DForOutWhenUnconnected=off
  wires:
  Aerodynamic Inputs/1 -> Bus Selector/1
  Bus Selector/1 -> [Alpha]  "<Alpha_perturbed>"
  Bus Selector/2 -> [Beta]  "<Beta_perturbed>"
  Bus Selector/3 -> [Q]  "<Q>"
  [Alpha] -> CL(AvsBvsM)/1
  [Beta] -> CL(AvsBvsM)/2
  [Mach] -> CL(AvsBvsM)/3
  Sum/1 -> CL/1
  CL(AvsBvsM)/1 -> Sum/1
  CL(Q)/1 -> Product/3
  Bus Selector/4 -> [Velocity]  "<Velocity_perturbed>"
  Product4/1 -> Sqrt/1
  Air/1 -> Product4/1
  Temperature (Kelvin)/1 -> Product4/3
  Gas Constant/1 -> Product4/2
  Sqrt/1 -> Divide/2
  Divide/1 -> [Mach]
  [Velocity] -> Divide/1
  [Alpha] -> CL(Q)/1
  Product/1 -> Sum/2
  [Q] -> Product/2
  Constant/1 -> Divide1/1
  [Velocity] -> Divide1/2
  Divide1/1 -> Product/1

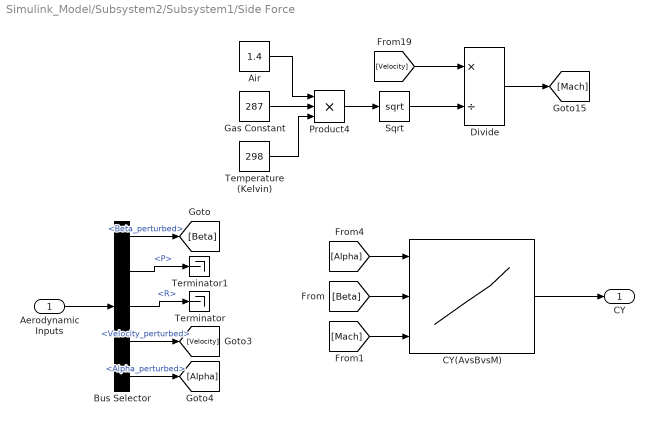
== system Simulink_Model/Subsystem2/Subsystem1/Side Force ==
  Aerodynamic Inputs : Inport
  Air : Constant  Value=1.4
  Bus Selector : BusSelector  OutputSignals=Beta_perturbed,P,R,Velocity_perturbed,Alpha_perturbed
  CY(AvsBvsM) : Lookup_n-D  NumberOfTableDimensions=3  BreakpointsForDimension1=[deg2rad(aoa(1)), deg2rad(aoa(2)), deg2rad(aoa(3)), deg2rad(aoa(4)), deg2rad(aoa(5))]  BreakpointsForDimension2=[deg2rad(ss(1)), deg2rad(ss(2)), deg2rad(ss(3)), deg2rad(ss(4))]  BreakpointsForDimension3=[mach(1), mach(2), mach(3), mach(4), mach(5)]  Table=-rocketAeroDatabase.side.CY  InternalRulePriority=Speed  RndMeth=Simplest
      settings: InputPortMap=u0,u1,u2
  Divide : Product  Inputs=*/
  Gas Constant : Constant  Value=287
  Product4 : Product  Inputs=3
  Sqrt : Sqrt
  Temperature (Kelvin) : Constant  Value=298
  Terminator : Terminator
  Terminator1 : Terminator
  CY : Outport  VectorParamsAs1DForOutWhenUnconnected=off
  wires:
  Aerodynamic Inputs/1 -> Bus Selector/1
  Bus Selector/1 -> [Beta]  "<Beta_perturbed>"
  Bus Selector/2 -> Terminator1/1  "<P>"
  Bus Selector/3 -> Terminator/1  "<R>"
  [Beta] -> CY(AvsBvsM)/2
  [Mach] -> CY(AvsBvsM)/3
  CY(AvsBvsM)/1 -> CY/1
  Bus Selector/4 -> [Velocity]  "<Velocity_perturbed>"
  Product4/1 -> Sqrt/1
  Air/1 -> Product4/1
  Temperature (Kelvin)/1 -> Product4/3
  Gas Constant/1 -> Product4/2
  Sqrt/1 -> Divide/2
  Divide/1 -> [Mach]
  [Velocity] -> Divide/1
  Bus Selector/5 -> [Alpha]  "<Alpha_perturbed>"
  [Alpha] -> CY(AvsBvsM)/1

== matlab function Simulink_Model/Equations of Motion 1/Equations of Motion ==
  data: Forces input size=3; statesDer output size=15; States input size=19; u1 input size=1; u2 input; T input; Time input size=1; A output; B1 output; B2 output; Moments input size=3; gamma output
function [statesDer,A,B1,B2,gamma] = fcn(Forces, States,u1,u2,T,Time, Moments)

%% states
Alpha = States(1);
Beta = States(2);
Theta = States(3);
Phi = States(4);
Psi = States(5);
Q = States(6);
P = States(7);
R = States(8);
Altitude = States(9);
Velocity = States(10);
North = States(11);
East = States(12);
Mass = States(13);
Inertia = States(14);
CG = States(15);
U = States(16);
V = States(17);
W = States(18);
d = States(19);

%% control inputs [rad]
if Time < 30
dYaw = 0;
dThe1 = u1;
dThe2 = u2;
else
dYaw = 0;
dThe1 = 0;
dThe2 = 0;
T=0;
end
% 
% if Time > 10
% e1 = 5;
% d1 =0;
% else
% e1=0;
% d1 =1;
% end

%%
Velocity = sqrt(U^2 + V^2 + W^2);
Alpha = atan(W/U);
Beta = asin(V/Velocity);

%% Thrust Vector Control
xcg = 3.5 - CG;

%% Upper Engine
ROT_UP = [cos(dThe1)*cos(dYaw) -cos(dThe1)*sin(dYaw) sin(dThe1);
       sin(dYaw)   cos(dYaw)   0 ;
       -sin(dThe1)*cos(dYaw)  sin(dThe1)*sin(dYaw)    cos(dThe1)];
F_up = ROT_UP'*[T/2 0 0]'; % for each engine 3by1 thrust of each engine...
r_up = [xcg 0 0.05];
M_up = cross(r_up,F_up);


%% Lower Engine
ROT_LOW = [cos(dThe2)*cos(dYaw) -cos(dThe2)*sin(dYaw) sin(dThe2);
       sin(dYaw)   cos(dYaw)   0 ;
       -sin(dThe2)*cos(dYaw)  sin(dThe2)*sin(dYaw)    cos(dThe2)];
F_low = ROT_LOW'*[T/2 0 0]'; % for each engine 3by1 thrust of each engine...
r_low = [xcg 0 -0.05];
M_low = cross(r_low,F_low);

%% Total Force and Moment on the Rocket Body
F_total = [F_up(1) + F_low(1) ;F_up(2) + F_low(2);F_up(3)+F_low(3)];
M_total = [M_up(1) + M_low(1) ;M_up(2) + M_low(2);M_up(3)+M_low(3)];
 
TVC = [F_total;M_total ];


% %% Thrust with deflections
% ROT = [cos(dThe)*cos(dYaw) -cos(dThe)*sin(dYaw) sin(dThe);
%        sin(dYaw)   cos(dYaw)   0 ;
%        -sin(dThe)*cos(dYaw)  sin(dThe)*sin(dYaw)    cos(dThe)];
%              
% F_ei = ROT'*[T 0 0]'; % for each engine 3by1 thrust of each engine...
% % Thrust in the engine own axes
% F_e = [F_ei(1) , F_ei(2) , F_ei(3)]'; % force vector from engine-i in body axes
% 
% r_e = [
%   xcg 0 0;
%  ]; 
% F = F_ei';
% M_ei = cross(r_e,F);
%  
% M_e = [sum(M_ei(:,1)), sum(M_ei(:,2)), sum(M_ei(:,3))]';
%  
% TVC = [F_e;M_e ];


%% Mass and Inertia Parameters
Gravity = 9.80665*(6371020/(6371020+Altitude))^2;

% Ixx = 0.58; % kg*m^2
Ixx = 1.08; % kg*m^2
Iyy = Inertia; %Inertia(2); % kg*m^2
Izz = Inertia; %Inertia(3); % kg*m^2 
Ixz = 0;
Iyz = 0;
Ixy = 0;

xCG = CG; % m
yCG = 0; % m
zCG = 0; % m

xRef = 3.5; % m
yRef = 0; % m
zRef = 0; % m

% FORCES

Lift = Forces(1);
Drag = Forces(2);
Side = Forces(3);

forceWindAxes = [-Drag; Side; -Lift];

transformMatrix = [cos(Alpha)*cos(Beta) sin(Beta) sin(Alpha)*cos(Beta); ...
                    -cos(Alpha)*sin(Beta) cos(Beta) -sin(Alpha)*sin(Beta); ...
                    -sin(Alpha) 0 cos(Alpha)];

forceBodyAxes = inv(transformMatrix)*forceWindAxes;

XA = forceBodyAxes(1);
YA = forceBodyAxes(2);
ZA = forceBodyAxes(3);


%% TVC
XT = TVC(1);
YT = TVC(2);
ZT = TVC(3);

MTX =  TVC(4);
MTY =  TVC(5);
MTZ =  TVC(6);

% MOMENTS

pitchingMomentREF = Moments(1);
rollingMomentREF = Moments(2);
yawingMomentREF = Moments(3);

distX = -(xCG - xRef); % m
distY = yCG - yRef; % m
distZ = -(zCG - zRef); % m

% pitchingMoment = pitchingMomentREF + ZA*distX + XA*distZ + XT*distZ +MTX ;
pitchingMoment = pitchingMomentREF + ZA*distX ;
% rollingMoment = rollingMomentREF + YA*distZ - ZA*distY + MTY;
rollingMoment = rollingMomentREF ;
% yawingMoment = yawingMomentREF + XA*distY - YA*distX + MTZ;
yawingMoment = yawingMomentREF - YA*distX;

%% EQUATIONS OF MOTION

UDot = R*V - Q*W - Gravity*sin(Theta) + (XA + XT)/Mass;
VDot = -R*U + P*W + Gravity*sin(Phi)*cos(Theta) + (YA + YT)/Mass;
WDot = Q*U - P*V + Gravity*cos(Phi)*cos(Theta) + (ZA + ZT)/Mass;


Ixz = 0;
F = Ixx*Izz - Ixz^2;
PDot = (Ixz*(Ixx-Iyy+Izz)*P*Q - (Izz*(Izz-Iyy)+Ixz^2)*Q*R + Izz*rollingMoment + Ixz*yawingMoment)/F;
QDot = ((Izz-Ixx)*P*R - Ixz*(R^2 - P^2) + pitchingMoment)/Iyy + MTY/Iyy;
RDot = ((Ixx*(Ixx-Iyy)+Ixz^2)*P*Q - Ixz*(Ixx-Iyy+Izz)*Q*R + Ixz*rollingMoment + Ixx*yawingMoment)/F +  + MTZ/F;

% KINEMATIC EQUATIONS
PhiDot = P + tan(Theta) * (Q*sin(Phi) + R*cos(Phi));
ThetaDot = Q*cos(Phi) - R*sin(Phi);
PsiDot = (Q*sin(Phi) + R*cos(Phi))/cos(Theta);

        
        
% NAVIGATION EQUATIONS

NorthDot = U*cos(Theta)*cos(Psi) + V*(-cos(Phi)*sin(Psi) + sin(Phi)*sin(Theta)*cos(Psi)) ...
    + W*(sin(Phi)*sin(Psi)+cos(Phi)*sin(Theta)*cos(Psi));

EastDot = U*cos(Theta)*sin(Psi) +  V*(cos(Phi)*cos(Psi) + sin(Phi)*sin(Theta)*sin(Psi)) ...
    + W*(-sin(Phi)*cos(Psi) + cos(Phi)*sin(Theta)*sin(Psi));

AltitudeDot = U*sin(Theta) - V*sin(Phi)*cos(Theta) - W*cos(Phi)*cos(Theta);

% Auxiliary 

VelocityDot = (U*UDot + V*VDot + W*WDot)/(Velocity);
AlphaDot = (U*WDot - W*UDot)/(U^2 + W^2);
BetaDot = (VDot*Velocity - V*VelocityDot)/(Velocity*sqrt(Velocity^2-V^2));

% AlphaDot = (-Lift - XT*sin(Alpha))/(Mass*Velocity*cos(Beta)) + Gravity*(cos(Theta)*cos(Phi)*cos(Alpha)...
%    + sin(Theta)*sin(Alpha))/(Velocity*cos(Beta)) + Q - tan(Beta)*(P*cos(Alpha) + R*sin(Alpha));
% 
% BetaDot = (Drag*sin(Beta) + Side*cos(Beta) - XT*cos(Alpha)*sin(Beta))/(Mass*Velocity)...
%     + Gravity*(sin(Theta)*cos(Alpha)*sin(Beta) + cos(Theta)*sin(Phi)*cos(Beta)...
%     - cos(Theta)*cos(Phi)*sin(Alpha)*sin(Beta))/Velocity + P*sin(Alpha) - R*cos(Alpha);
% 
% VelocityDot = (-Drag*cos(Beta) + Side*sin(Beta) + XT*cos(Alpha)*cos(Beta))/Mass + ...
%                 Gravity*(-sin(Theta)*cos(Alpha)*cos(Beta) +...
%                 cos(Theta)*sin(Phi)*sin(Beta) + cos(Theta)*cos(Phi)*sin(Alpha)*cos(Beta));
% 
% if Time < 5.17
%     MassDot = -3.6; % kg/s
%     cgDot = -0.031; % m/s
%     InertiaDot = -3.3; % kg.m^2/s
% else
%     MassDot = 0; % kg/s
%     cgDot = 0; % m/s
%     InertiaDot = 0; % kg.m^2/s    
% end

if Time < 31
    MassDot = -3.6; % kg/s
    cgDot = -0.031; % m/s
    InertiaDot = -3.3; % kg.m^2/s
else
    MassDot = 0; % kg/s
    cgDot = 0; % m/s
    InertiaDot = 0; % kg.m^2/s    
end


statesDer = [AlphaDot; BetaDot; ThetaDot; PhiDot; PsiDot; QDot; PDot; RDot; AltitudeDot;...
            VelocityDot; NorthDot; EastDot; MassDot; InertiaDot; cgDot];
gamma = Theta ;
    

% %% Actuator Health Parameters
% if Time > 10
% d1 = 1;
% e1 = deg2rad(0);
% else
% d1 = 1;
% e1 = 0;
% end

% D = [d1 0 ;
%      0  1];
% 
% % E = [e1 0 ]';

%% NDI FEEDBACK LINEARIZATION
% Pitch rate
% Pitch rate
if Time < 30
% A = ((Izz-Ixx)*P*R - Ixz*(R^2 - P^2) + pitchingMoment)/Iyy + MTY/Iyy;
A = ((Izz-Ixx)*P*R - Ixz*(R^2 - P^2) + pitchingMoment)/Iyy;
invB = pinv([(-T/2*xcg/Iyy )*d;-T/2*xcg/Iyy]); 
%invB = pinv([-T/2*xcg/Iyy*d1 ;-T/2*xcg/Iyy]);
B1  = invB(1,1);
B2  = invB(1,2);

else
A = 1;
B1 = 1;
B2 = 1;

end
% if Time < 31
% A = ((Izz-Ixx)*P*R - Ixz*(R^2 - P^2) + pitchingMoment)/Iyy + MTY/Iyy;
% B = inv(-T/2*xcg/Iyy); 
% else
%     A = 1;
%     B = 1;
% end
% Yaw rate
% RDot = ((Ixx*(Ixx-Iyy)+Ixz^2)*P*Q - Ixz*(Ixx-Iyy+Izz)*Q*R + Ixz*rollingMoment + Ixx*yawingMoment)/F + MTZ/F;
% if Time < 30
% A = ((Ixx*(Ixx-Iyy))*P*Q + Ixx*yawingMoment)/F + MTZ/F
% B = inv(T*xcg/F)
% else
% A = 1;
% B = 1;
% end

== matlab function Simulink_Model/Equations of Motion 1/Predict loss of effectiveness ==
  data: x input; y_pred output; time input



function y_pred = fcn(x,time)

% coder.extrinsic('py.predictorModule.run')

y_pred = 1;
% y_pred = double(py.predictorModule.run(x));

if time >5.2 && time < 30

 y_pred = double(py.predictorModule.run(x));

    else
        y_pred = 1;
        
end

end
